simulink model "flyback"  (R2018a)
settings: Solver=VariableStepAuto  StartTime=0.0  StopTime=0.1  MaxStep=1e-7  RelTol=1e-3
libraries: powerlib x13, powerlib_meascontrol x1
settings Model: Creator=DELL  LastModifiedBy=DELL

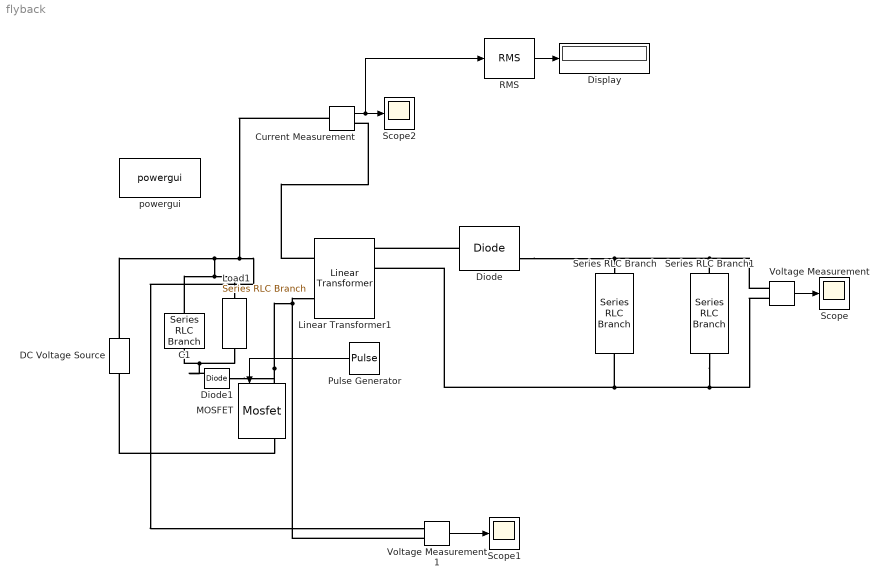
== system flyback ==
  C1 : powerlib/Elements/Series RLC Branch  LConnTagsString=__new0  RConnTagsString=__new0  BranchType=C  Resistance=1e-4  Inductance=200e-6  SetiL0=off  InitialCurrent=0  Capacitance=47e-6  Setx0=off  InitialVoltage=0  Measurements=None
  Current Measurement : powerlib/Measurements/Current Measurement  PhasorSimulation=off  OutputType=Complex  PSBequivalent=0
  DC Voltage Source : powerlib/Electrical Sources/DC Voltage Source  Amplitude=36  Measurements=None
  Diode : powerlib/Power Electronics/Diode  Ron=0.001  Lon=0  Vf=0.8  IC=0  UseSnubber=0  Rs=500  Cs=250e-9  Measurements=on
  Diode1 : powerlib/Power Electronics/Diode  Ron=0.001  Lon=0  Vf=0.8  IC=0  UseSnubber=0  Rs=500  Cs=250e-9  Measurements=on
  Display : Display
  Linear Transformer1 : powerlib/Elements/Linear Transformer  UNITS=SI  NominalPower=[ 400 50000 ]  winding1=[16 0.080 1.65e-6]  winding2=[10 0.080 1.65e-6]  ThreeWindings=on  winding3=[16 0.080 1.65e-6]  RmLm=[1.0805e+06 20e-6]  Measurements=All voltages and currents  DataType=on
  Load1 : powerlib/Elements/Series RLC Branch  LConnTagsString=__new0  RConnTagsString=__new0  BranchType=R  Resistance=440  Inductance=200e-6  SetiL0=off  InitialCurrent=0  Capacitance=400e-6  Setx0=off  InitialVoltage=0  Measurements=Branch current
  MOSFET : powerlib/Power Electronics/Mosfet  Ron=1e-3  Lon=0  Rd=1e-3  Vfd=0  IC=0  Rs=1e6  Cs=inf  Measurements=on
  Pulse Generator : DiscretePulseGenerator  PulseType=Time based  Period=1/45e3  PulseWidth=45
  RMS : powerlib_meascontrol/Measurements/RMS  TrueRMS=on  Freq=45000  RMSInit=120  Ts=0
  Scope : Scope
  Scope1 : Scope
  Scope2 : Scope
  Series RLC Branch : powerlib/Elements/Series RLC Branch  LConnTagsString=__new0  RConnTagsString=__new0  BranchType=RLC  Resistance=0.02  Inductance=0  SetiL0=off  InitialCurrent=0  Capacitance=820e-6  Setx0=off  InitialVoltage=0  Measurements=None
  Series RLC Branch1 : powerlib/Elements/Series RLC Branch  LConnTagsString=__new0  RConnTagsString=__new0  BranchType=R  Resistance=15^2/60  Inductance=0  SetiL0=off  InitialCurrent=0  Capacitance=0  Setx0=off  InitialVoltage=0  Measurements=None
  Voltage Measurement : powerlib/Measurements/Voltage Measurement  PhasorSimulation=off  OutputType=Complex  PSBequivalent=0
  Voltage Measurement1 : powerlib/Measurements/Voltage Measurement  PhasorSimulation=off  OutputType=Complex  PSBequivalent=0
  powergui : powerlib/powergui  Priority=1  SimulationMode=Continuous  SampleTime=50e-6  frequency=60  Iterations=50  frequencyindice=0  Pbase=100e6  ErrMax=1e-4  UnitsV=kV  UnitsW=MW  buscounter=0  FunctionMessages=off  echomessages=off  EnableUseOfTLC=off  CurrentSourceSwitches=off  DisableSnubberDevices=off  DisableRonSwitches=off  DisableVfSwitches=off  DisplayEquations=off  SolverType=Tustin/Backward Euler (TBE)  Interpol=off  ExternalGateDelay=off  methode=off  Ts=100  x0status=blocks  SPID=on  SwTol=0  HookPort=off  RestoreLinks=warning  ResistiveCurrentMeasurement=off  Frange=[0:2:500]  Ylog=off  Xlog=on  ShowGrid=off  save=off  variable=ZData  structure=0  ZoomFFT=off  StartTime=0.0  cycles=1  DisplayStyle=1  fundamental=60  FreqAxis=off  MaxFrequency=1000  frequencyindicesteady=1  RmsSteady=1  display=off
  wires:
  Pulse Generator/1 -> MOSFET/1
  Voltage Measurement/1 -> Scope/1
  Voltage Measurement1/1 -> Scope1/1
  Current Measurement/1 -> RMS/1, Scope2/1
  RMS/1 -> Display/1
  connections:
  MOSFET/RConn1 -- DC Voltage Source/LConn1
  Diode/LConn1 -- Linear Transformer1/RConn1
  Diode/RConn1 -- Voltage Measurement/LConn1 -- Series RLC Branch1/LConn1 -- Series RLC Branch/LConn1
  Series RLC Branch/RConn1 -- Linear Transformer1/RConn2 -- Voltage Measurement/LConn2 -- Series RLC Branch1/RConn1
  Load1/LConn1 -- Diode1/RConn1 -- C1/LConn1
  DC Voltage Source/RConn1 -- C1/RConn1 -- Load1/RConn1 -- Current Measurement/LConn1 -- Voltage Measurement1/LConn1
  Linear Transformer1/LConn1 -- Current Measurement/RConn1
  Voltage Measurement1/LConn2 -- Diode1/LConn1 -- MOSFET/LConn1 -- Linear Transformer1/LConn2
